simulink model "kinsim_2link_planar"  (R2020a)
settings: Solver=ode3  StartTime=0.0  StopTime=10.0  FixedStep=0.05  RelTol=1e-3
values from neighbouring files (symbols this model uses):
  L1 = 0.337    [dynsim_test_urdf_init.m]    (also in init_2link_planar.m)
  L2 = 0.210    (= 0.21)    [dynsim_test_urdf_init.m]    (also in init_2link_planar.m)
  L3 = 0.268    [dynsim_test_urdf_init.m]    (also in init_2link_planar.m)
  L4 = 0    [dynsim_test_urdf_init.m]    (also in init_2link_planar.m)
  L5 = 0.174    [dynsim_test_urdf_init.m]    (also in init_2link_planar.m)
  L6 = 0    [dynsim_test_urdf_init.m]    (also in init_2link_planar.m)
libraries: robotlib x12
settings Model: Creator=bascetta  LastModifiedBy=sofia
settings OptimizationCC: EnhancedBackFolding=on  PassReuseOutputArgsAs=Individual arguments  ZeroExternalMemoryAtStartup=off  ZeroInternalMemoryAtStartup=off  MaxStackSize=64  OptimizeBlockOrder=speed  DifferentSizesBufferReuse=on  OptimizationCustomize=off  EfficientTunableParamExpr=on
settings DebuggingCC: ParameterTunabilityLossMsg=error
settings HardwareCC: ProdBitPerPointer=32  ProdBitPerSizeT=32  ProdBitPerPtrDiffT=32  ProdLargestAtomicFloat=None  ProdIntDivRoundTo=Undefined  ProdEndianess=Unspecified  ProdWordSize=32  ProdHWDeviceType=Generic->Unspecified (assume 32-bit Generic)
settings RTWCC: SystemTargetFile=ert.tlc  HardwareBoard=Robot Operating System (ROS)  TemplateMakefile=ert_default_tmf  GenerateReport=on  Toolchain=Catkin  IncludeHyperlinkInReport=on  LaunchReport=on  TargetLang=C++  GenerateTraceInfo=on  GenerateTraceReport=on  GenerateTraceReportSl=on  GenerateTraceReportSf=on  GenerateTraceReportEml=on
settings CodeAppCC: ForceParamTrailComments=on  IgnoreCustomStorageClasses=off  OperatorAnnotations=on  SimulinkDataObjDesc=on  SFDataObjDesc=on  InsertBlockDesc=on
settings ERTTargetCC: SupportContinuousTime=on  SupportVariableSizeSignals=on

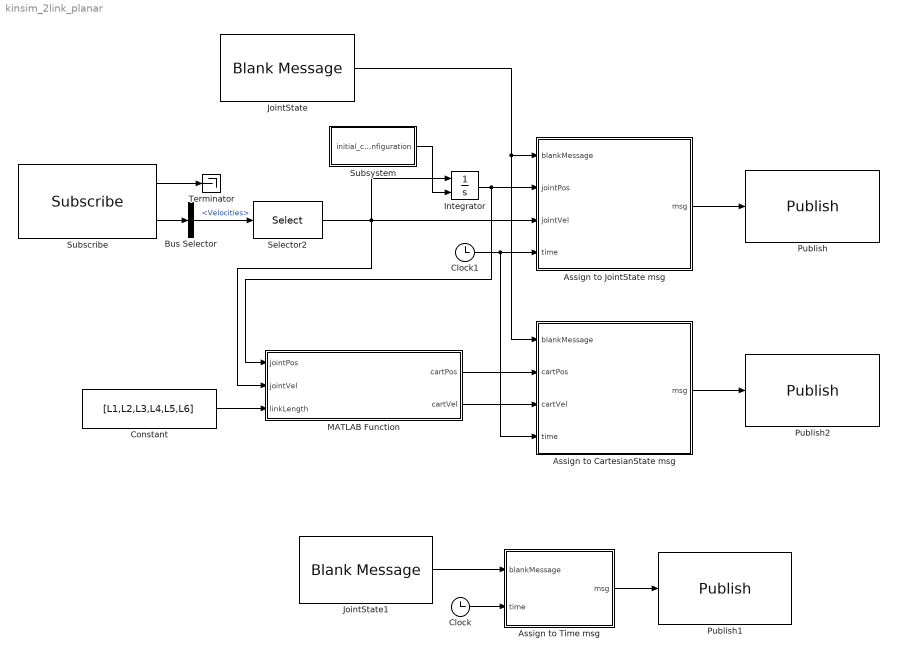
== system kinsim_2link_planar ==
  Assign to CartesianState msg : MATLAB Function  TreatAsAtomicUnit=on
  Assign to JointState msg : MATLAB Function  TreatAsAtomicUnit=on
  Assign to Time msg : MATLAB Function  TreatAsAtomicUnit=on
  Bus Selector : BusSelector  OutputSignals=Velocities
  Clock : Clock
  Clock1 : Clock
  Constant : Constant  Value=[L1,L2,L3,L4,L5,L6]
  Integrator : Integrator  InitialConditionSource=external  InitialCondition=[0,0]
  JointState : robotlib/Blank Message  messageClass=Message  entityType=sensor_msgs/JointState  messageType=sensor_msgs/JointState  SampleTime=inf
  JointState1 : robotlib/Blank Message  messageClass=Message  entityType=rosgraph_msgs/Clock  messageType=rosgraph_msgs/Clock  SampleTime=inf
  MATLAB Function : MATLAB Function  TreatAsAtomicUnit=on
  Publish : robotlib/Publish  topicSource=Specify your own  topic=/edo/joint_states  messageType=sensor_msgs/JointState  messageQueueLength=1
  Publish1 : robotlib/Publish  topicSource=Specify your own  topic=/clock  messageType=rosgraph_msgs/Clock  messageQueueLength=1
  Publish2 : robotlib/Publish  topicSource=Specify your own  topic=/cartesian_states  messageType=sensor_msgs/JointState  messageQueueLength=1
  Selector2 : Selector  IndexOptions=Starting index (dialog)  Indices=[2]  OutputSizes=6
  Subscribe : robotlib/Subscribe  topicSource=Specify your own  topic=/joint_trajectory  messageType=trajectory_msgs/JointTrajectoryPoint  sampleTime=-1  messageQueueLength=1
  Subsystem : Subsystem
  Terminator : Terminator
  wires:
  Subscribe/1 -> Terminator/1
  Subscribe/2 -> Bus Selector/1
  Bus Selector/1 -> Selector2/1  "<Velocities>"
  Integrator/1 -> MATLAB Function/1(jointPos), Assign to JointState msg/2(jointPos)
  Selector2/1 -> Assign to JointState msg/3(jointVel), MATLAB Function/2(jointVel), Integrator/1
  Assign to JointState msg/1(msg) -> Publish/1
  JointState/1 -> Assign to CartesianState msg/1(blankMessage), Assign to JointState msg/1(blankMessage)
  JointState1/1 -> Assign to Time msg/1(blankMessage)
  Clock/1 -> Assign to Time msg/2(time)
  Assign to Time msg/1(msg) -> Publish1/1
  Clock1/1 -> Assign to CartesianState msg/4(time), Assign to JointState msg/4(time)
  Subsystem/1(initial_configuration) -> Integrator/2
  MATLAB Function/1(cartPos) -> Assign to CartesianState msg/2(cartPos)
  MATLAB Function/2(cartVel) -> Assign to CartesianState msg/3(cartVel)
  Assign to CartesianState msg/1(msg) -> Publish2/1
  Constant/1 -> MATLAB Function/3(linkLength)

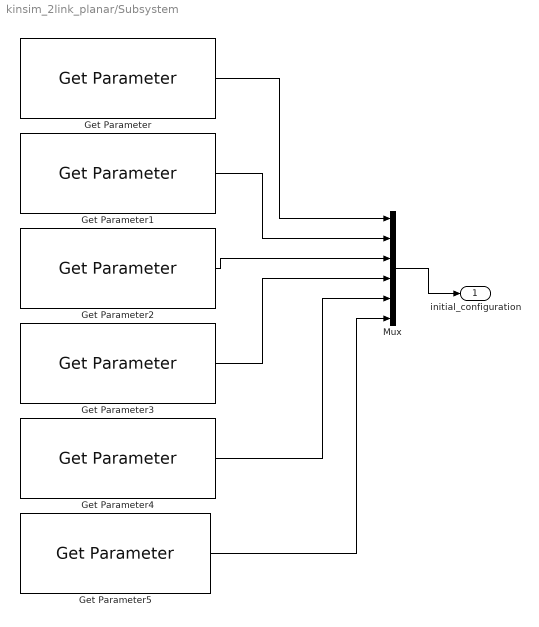
== system kinsim_2link_planar/Subsystem ==
  Get Parameter : robotlib/Get Parameter  ParameterSource=Specify your own  ParameterName=/kinsim_2link_planar/q1_initial  ParameterType=double  ParameterMaxArrayLength=16  ParameterInitialValue=0  SampleTime=-1  ShowErrorCodeOutput=off  ModelName=kinsim_2link_planar  BlockId=ParamGet_kinsim_2link_planar_61
      settings: SourceProductBaseCode=RR
  Get Parameter1 : robotlib/Get Parameter  ParameterSource=Specify your own  ParameterName=/kinsim_2link_planar/q2_initial  ParameterType=double  ParameterMaxArrayLength=16  ParameterInitialValue=0  SampleTime=-1  ShowErrorCodeOutput=off  ModelName=kinsim_2link_planar  BlockId=ParamGet_kinsim_2link_planar_65
      settings: SourceProductBaseCode=RR
  Get Parameter2 : robotlib/Get Parameter  ParameterSource=Specify your own  ParameterName=/kinsim_2link_planar/q3_initial  ParameterType=double  ParameterMaxArrayLength=16  ParameterInitialValue=0  SampleTime=-1  ShowErrorCodeOutput=off  ModelName=kinsim_2link_planar  BlockId=ParamGet_kinsim_2link_planar_81
      settings: SourceProductBaseCode=RR
  Get Parameter3 : robotlib/Get Parameter  ParameterSource=Specify your own  ParameterName=/kinsim_2link_planar/q4_initial  ParameterType=double  ParameterMaxArrayLength=16  ParameterInitialValue=0.0  SampleTime=-1  ShowErrorCodeOutput=off  ModelName=kinsim_2link_planar  BlockId=ParamGet_kinsim_2link_planar_82
      settings: SourceProductBaseCode=RR
  Get Parameter4 : robotlib/Get Parameter  ParameterSource=Specify your own  ParameterName=/kinsim_2link_planar/q5_initial  ParameterType=double  ParameterMaxArrayLength=16  ParameterInitialValue=0.0  SampleTime=-1  ShowErrorCodeOutput=off  ModelName=kinsim_2link_planar  BlockId=ParamGet_kinsim_2link_planar_83
      settings: SourceProductBaseCode=RR
  Get Parameter5 : robotlib/Get Parameter  ParameterSource=Specify your own  ParameterName=/kinsim_2link_planar/q6_initial  ParameterType=double  ParameterMaxArrayLength=16  ParameterInitialValue=0.0  SampleTime=-1  ShowErrorCodeOutput=off  ModelName=kinsim_2link_planar  BlockId=ParamGet_kinsim_2link_planar_84
      settings: SourceProductBaseCode=RR
  Mux : Mux  Inputs=6
  initial_configuration : Outport
  wires:
  Mux/1 -> initial_configuration/1
  Get Parameter/1 -> Mux/1
  Get Parameter1/1 -> Mux/2
  Get Parameter2/1 -> Mux/3
  Get Parameter3/1 -> Mux/4
  Get Parameter4/1 -> Mux/5
  Get Parameter5/1 -> Mux/6

== matlab function kinsim_2link_planar/Assign to Time msg ==
  data: blankMessage input Bus: SL_Bus_kinsim_2link_planar_rosgraph_msgs_Clock; msg output Bus: SL_Bus_kinsim_2link_planar_rosgraph_msgs_Clock; time input
function msg = assign_Time(blankMessage,time)
%#codegen

% Assign the output message to be the same with input blank message
msg = blankMessage;

% Convert and set time
msg.Clock_.Sec  = fix(time);
msg.Clock_.Nsec = fix((time-fix(time))*1e9);

== matlab function kinsim_2link_planar/Assign to JointState msg ==
  data: blankMessage input; msg output Bus: SL_Bus_kinsim_2link_planar_sensor_msgs_JointState; jointPos input; jointVel input; time input
function msg = assign_JointState(blankMessage,jointPos,jointVel,time)
%#codegen

% Assign the output message to be the same with input blank message
msg = blankMessage;

% Initialize time stamp
msg.Header.Stamp.Sec  = fix(time);
msg.Header.Stamp.Nsec = fix((time-fix(time))*1e9);

% Set the number of strings in the string array, and joint positions/velocities in the position/velocity array
numJoints = length(jointPos);
msg.Name_SL_Info.CurrentLength = uint32(numJoints);
msg.Position_SL_Info.CurrentLength = uint32(numJoints);
msg.Velocity_SL_Info.CurrentLength = uint32(numJoints);

% Set the individual components in the message arrays
strArrayToAssign = {'edo_joint_1', 'edo_joint_2', 'edo_joint_3', 'edo_joint_4', 'edo_joint_5', 'edo_joint_6'};

for idx=1:numJoints
    str = strArrayToAssign{idx};
    strLength = length(str);
    msg.Name(idx).Data(1:strLength) = uint8(str);
    msg.Name(idx).Data_SL_Info.CurrentLength = uint32(strLength);

    msg.Position(idx) = jointPos(idx);
    msg.Velocity(idx) = jointVel(idx);
end

== matlab function kinsim_2link_planar/MATLAB Function ==
  data: jointPos input; cartPos output; jointVel input; cartVel output; linkLength input
function [cartPos, cartVel] = forward_kinematics_2link(jointPos,jointVel,linkLength)

cartPos = zeros(1,2);
cartVel = zeros(1,2);

L1 = linkLength(1);
L2 = linkLength(2);
L3 = linkLength(3);
L4 = linkLength(4);
L5 = linkLength(5);
L6 = linkLength(6);
q1 = jointPos(1);
q2 = jointPos(2);
q3 = jointPos(3);
q4 = jointPos(4);
q5 = jointPos(5);
q6 = jointPos(6);
qv1 = jointVel(1);
qv2 = jointVel(2);
qv3 = jointVel(3);
qv4 = jointVel(4);
qv5 = jointVel(5);
qv6 = jointVel(6);

cartPos(1) = L1*cos(q1)+L2*cos(q1+q2)+L3*cos(q1+q2+q3)+L4*cos(q1+q2+q3+q4)+L5*cos(q1+q2+q3+q4+q5)+L6*cos(q1+q2+q3+q4+q5+q6);
cartPos(2) = L1*sin(q1)+L2*sin(q1+q2)+L3*sin(q1+q2+q3)+L4*sin(q1+q2+q3+q4)+L5*sin(q1+q2+q3+q4+q5)+L6*sin(q1+q2+q3+q4+q5+q6);
cartVel(1) = -L1*qv1*sin(q1)-L2*(qv1+qv2)*sin(q1+q2)-L3*(qv1+qv2+qv3)*sin(q1+q2+q3)-L4*(qv1+qv2+qv3+qv4)*sin(q1+q2+q3+q4)-L5*(qv1+qv2+qv3+qv4+qv5)*sin(q1+q2+q3+q4+q5)-L6*(qv1+qv2+qv3+qv4+qv5+qv6)*sin(q1+q2+q3+q4+q5+q6);
cartVel(2) = L1*qv1*cos(q1)+L2*(qv1+qv2)*cos(q1+q2)+L3*(qv1+qv2+qv3)*cos(q1+q2+q3)+L4*(qv1+qv2+qv3+qv4)*cos(q1+q2+q3+q4)+L5*(qv1+qv2+qv3+qv4+qv5)*cos(q1+q2+q3+q4+q5)+L6*(qv1+qv2+qv3+qv4+qv5+qv6)*cos(q1+q2+q3+q4+q5+q6);

== matlab function kinsim_2link_planar/Assign to CartesianState msg ==
  data: blankMessage input; msg output Bus: SL_Bus_kinsim_2link_planar_sensor_msgs_JointState; cartPos input; cartVel input; time input
function msg = assign_CartesianState(blankMessage,cartPos,cartVel,time)
%#codegen

% Assign the output message to be the same with input blank message
msg = blankMessage;

% Initialize time stamp
msg.Header.Stamp.Sec  = fix(time);
msg.Header.Stamp.Nsec = fix((time-fix(time))*1e9);

% Set the number of strings in the string array, and joint positions/velocities in the position/velocity array
numCoordinates = length(cartPos);
msg.Name_SL_Info.CurrentLength = uint32(numCoordinates);
msg.Position_SL_Info.CurrentLength = uint32(numCoordinates);
msg.Velocity_SL_Info.CurrentLength = uint32(numCoordinates);

% Set the individual components in the message arrays
strArrayToAssign = {'edo_joint_1', 'edo_joint_2', 'edo_joint_3', 'edo_joint_4', 'edo_joint_5', 'edo_joint_6'};

for idx=1:numCoordinates
    str = strArrayToAssign{idx};
    strLength = length(str);
    msg.Name(idx).Data(1:strLength) = uint8(str);
    msg.Name(idx).Data_SL_Info.CurrentLength = uint32(strLength);

    msg.Position(idx) = cartPos(idx);
    msg.Velocity(idx) = cartVel(idx);
end
